simulink model "deteccao_2016_V7_somenteEHAs_comfiltro_"  (R2016a)
settings: Solver=FixedStepAuto  StartTime=72.65  StopTime=73.9  FixedStep=Ts  MaxStep=1e-7  RelTol=1e-4  AbsTol=1e-4
PreLoadFcn:
  | % -- Recommended Settings --
  | %
  | %  Simulink:
  | %      Solver: Ode23t
  | %      Relative tolerance = 1e-3
  | %       Max step size = 0.2
  | %
  | %  Powergui:
  |          Ts = 1e-07; % (discrete electrical model)
  | %
  | %  Control systems:
  |          Ts_control = 10*Ts; % (discrete control system)
  | %
  | % ----------------------------------
undefined symbols (not defined in the file or in its folder): C, L, R1, R2, sigbuilder_block
libraries: powerlib x92, dsparch4 x12, simulink x6, sps_avr x1, powerlib_meascontrol x1
(part 1 of 2)
settings Model: Creator=Joao  LastModifiedBy=Joao
settings DataIOCC: FinalStateName=xFinal_400_fixedstep  InitialState=xFinal_400_fixedstep  LimitDataPoints=on  SaveCompleteFinalSimState=on
settings DebuggingCC: UnconnectedInputMsg=none  UnconnectedOutputMsg=none  UnconnectedLineMsg=none  AllowSymbolicDim=off
settings ConfigComp: CovModelRefEnable=Off  CovSFcnEnable=off

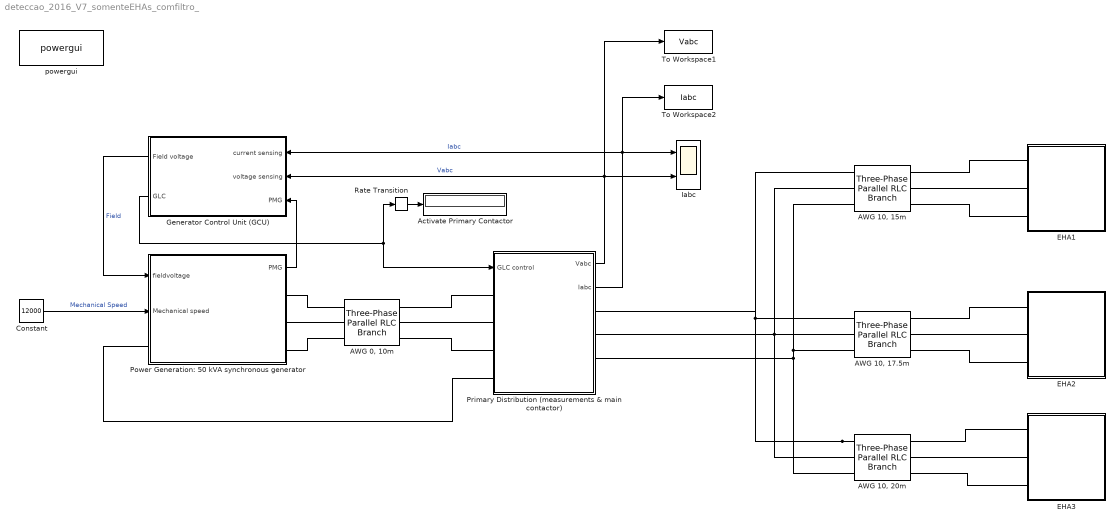
== system deteccao_2016_V7_somenteEHAs_comfiltro_ ==
  "AWG 0, 10m" : powerlib/Elements/Three-Phase Parallel RLC Branch  LConnTagsString=A|B|C  RConnTagsString=A|B|C  BranchType=RL  Resistance=0.00047*10  Inductance=0.2663e-06*10  Capacitance=0  Measurements=None
  "AWG 10, 15m" : powerlib/Elements/Three-Phase Parallel RLC Branch  LConnTagsString=A|B|C  RConnTagsString=A|B|C  BranchType=RL  Resistance=0.0036*15  Inductance=5.2869e-07*15  Capacitance=0  Measurements=None
  "AWG 10, 17.5m" : powerlib/Elements/Three-Phase Parallel RLC Branch  LConnTagsString=A|B|C  RConnTagsString=A|B|C  BranchType=RL  Resistance=0.0036*17.5  Inductance=5.2869e-07*17.5  Capacitance=0  Measurements=None
  "AWG 10, 20m" : powerlib/Elements/Three-Phase Parallel RLC Branch  LConnTagsString=A|B|C  RConnTagsString=A|B|C  BranchType=RL  Resistance=0.0036*20  Inductance=5.2869e-07*20  Capacitance=0  Measurements=None
  Activate Primary Contactor : Display
      settings: SampleTime=1e-2
  Constant : Constant  Value=12000
  EHA1 : Subsystem
  EHA2 : Subsystem
  EHA3 : Subsystem
  Generator Control Unit (GCU) : Subsystem
      mask Display: image(imread('power_aircraft_distribution_GCU.jpg','jpg'))
  Iabc : Scope  NumInputPorts=2
  Power Generation: 50 kVA synchronous generator : Subsystem
      mask Display: image(imread('power_aircraft_distribution_APU_Generator.jpg','jpg'))
  Primary Distribution (measurements & main contactor) : Subsystem
  Rate Transition : RateTransition  OutPortSampleTimeOpt=Inherit  OutPortSampleTime=Ts
  To Workspace1 : ToWorkspace  VariableName=Vabc  SaveFormat=Structure With Time  SampleTime=-1
  To Workspace2 : ToWorkspace  VariableName=Iabc  SaveFormat=Structure With Time  SampleTime=-1
  powergui : powerlib/powergui  Priority=1  SimulationMode=Continuous  SolverType=Tustin/Backward Euler (TBE)  SampleTime=Ts  frequency=60  SPID=on  DisableSnubberDevices=on  DisableRonSwitches=on  DisableVfSwitches=on  SwTol=0  DisplayEquations=off  Interpol=off  ExternalGateDelay=off  methode=off  Ts=100  FunctionMessages=on  echomessages=off  HookPort=off  EnableUseOfTLC=off  x0status=blocks  frequencyindice=0  Pbase=100e6  ErrMax=1e-4  Iterations=50  UnitsV=kV  UnitsW=MW  buscounter=0  RestoreLinks=warning  ResistiveCurrentMeasurement=off  Frange=[0:2:500]  Ylog=off  Xlog=on  ShowGrid=off  save=off  variable=ZData  structure=0  ZoomFFT=off  StartTime=0.0  cycles=1  DisplayStyle=1  fundamental=60  FreqAxis=off  MaxFrequency=1000  frequencyindicesteady=1  RmsSteady=1  display=off
  wires:
  Power Generation: 50 kVA synchronous generator/1(PMG) -> Generator Control Unit (GCU)/3(PMG)
  Generator Control Unit (GCU)/1(Field voltage) -> Power Generation: 50 kVA synchronous generator/1(fieldvoltage)  "Field"
  Primary Distribution (measurements & main contactor)/1(Vabc) -> Iabc/2, To Workspace1/1, Generator Control Unit (GCU)/2(voltage sensing)  "Vabc"
  Primary Distribution (measurements & main contactor)/2(Iabc) -> Generator Control Unit (GCU)/1(current sensing), To Workspace2/1, Iabc/1  "Iabc"
  Generator Control Unit (GCU)/2(GLC) -> Primary Distribution (measurements & main contactor)/1(GLC control), Rate Transition/1
  Constant/1 -> Power Generation: 50 kVA synchronous generator/2(Mechanical speed)  "Mechanical Speed"
  Rate Transition/1 -> Activate Primary Contactor/1
  connections:
  "AWG 10, 20m"/LConn1 -- "AWG 10, 15m"/LConn1 -- Primary Distribution (measurements & main contactor)/RConn1 -- "AWG 10, 17.5m"/LConn1
  "AWG 10, 17.5m"/LConn3 -- "AWG 10, 15m"/LConn3 -- "AWG 10, 20m"/LConn3 -- Primary Distribution (measurements & main contactor)/RConn3
  "AWG 10, 17.5m"/LConn2 -- "AWG 10, 15m"/LConn2 -- Primary Distribution (measurements & main contactor)/RConn2 -- "AWG 10, 20m"/LConn2
  "AWG 0, 10m"/RConn2 -- Primary Distribution (measurements & main contactor)/LConn2
  "AWG 0, 10m"/LConn2 -- Power Generation: 50 kVA synchronous generator/RConn2
  "AWG 0, 10m"/LConn1 -- Power Generation: 50 kVA synchronous generator/RConn1
  "AWG 0, 10m"/LConn3 -- Power Generation: 50 kVA synchronous generator/RConn3
  "AWG 0, 10m"/RConn1 -- Primary Distribution (measurements & main contactor)/LConn1
  "AWG 0, 10m"/RConn3 -- Primary Distribution (measurements & main contactor)/LConn3
  Power Generation: 50 kVA synchronous generator/LConn1 -- Primary Distribution (measurements & main contactor)/LConn4
  "AWG 10, 15m"/RConn1 -- EHA1/LConn1
  "AWG 10, 15m"/RConn2 -- EHA1/LConn2
  "AWG 10, 15m"/RConn3 -- EHA1/LConn3
  "AWG 10, 17.5m"/RConn1 -- EHA2/LConn1
  "AWG 10, 17.5m"/RConn2 -- EHA2/LConn2
  "AWG 10, 17.5m"/RConn3 -- EHA2/LConn3
  EHA3/LConn1 -- "AWG 10, 20m"/RConn1
  EHA3/LConn2 -- "AWG 10, 20m"/RConn2
  "AWG 10, 20m"/RConn3 -- EHA3/LConn3

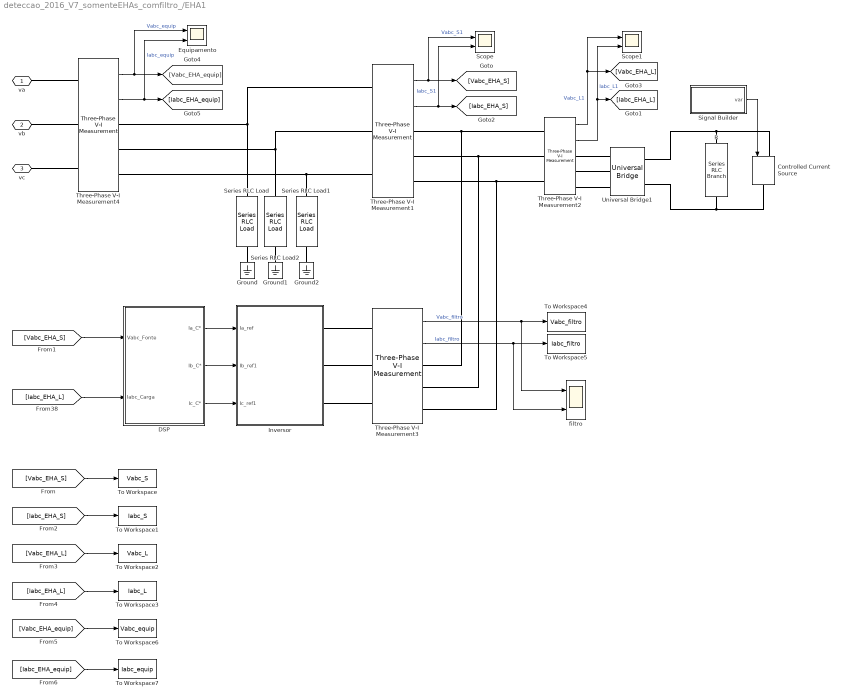
== system deteccao_2016_V7_somenteEHAs_comfiltro_/EHA1 ==
  Controlled Current Source : powerlib/Electrical Sources/Controlled Current Source  Initialize=on  Source_Type=AC  Amplitude=0  Phase=0  Frequency=0  Measurements=None
  DSP : Subsystem
  Equipamento : Scope  NumInputPorts=2
  Ground : powerlib/Elements/Ground  LConnTagsString=a
  Ground1 : powerlib/Elements/Ground  LConnTagsString=a
  Ground2 : powerlib/Elements/Ground  LConnTagsString=a
  Inversor : Subsystem
  R : powerlib/Elements/Series RLC Branch  LConnTagsString=__new0  RConnTagsString=__new0  BranchType=R  Resistance=10e3  Inductance=1e-3  SetiL0=off  InitialCurrent=0  Capacitance=1e-10  Setx0=off  InitialVoltage=0  Measurements=None
  Scope : Scope  NumInputPorts=2
  Scope1 : Scope  NumInputPorts=2
  Series RLC Load : powerlib/Elements/Series RLC Load  LConnTagsString=a  RConnTagsString=__new0  NominalVoltage=115  NominalFrequency=400  ActivePower=1  InductivePower=115^2*2*pi*400*C  CapacitivePower=0  Setx0=off  InitialVoltage=0  SetiL0=off  InitialCurrent=0  Measurements=None  LoadType=constant Z
  Series RLC Load1 : powerlib/Elements/Series RLC Load  LConnTagsString=a  RConnTagsString=__new0  NominalVoltage=115  NominalFrequency=400  ActivePower=1  InductivePower=115^2*2*pi*400*C  CapacitivePower=0  Setx0=off  InitialVoltage=0  SetiL0=off  InitialCurrent=0  Measurements=None  LoadType=constant Z
  Series RLC Load2 : powerlib/Elements/Series RLC Load  LConnTagsString=a  RConnTagsString=__new0  NominalVoltage=115  NominalFrequency=400  ActivePower=1  InductivePower=115^2*2*pi*400*C  CapacitivePower=0  Setx0=off  InitialVoltage=0  SetiL0=off  InitialCurrent=0  Measurements=None  LoadType=constant Z
  Signal Builder : Subsystem  Tag=STV Subsys  LoadFcn=sigbuilder_block('load');  StartFcn=sigbuilder_block('start');  StopFcn=sigbuilder_block('stop');  ClipboardFcn=sigbuilder_block('clipboard');  mask(Sigbuilder block){}
      mask help: Simulink:masks:SigbuilderBlock_MD
      mask init:
      | if ~strcmp(get_param(bdroot(gcbh),'SimulationStatus'),'stopped') tuvar = sigbuilder_block('maskInit'); end
      settings: CopyFcn=sigbuilder_block('copy');  DeleteFcn=sigbuilder_block('delete');  ModelCloseFcn=sigbuilder_block('modelClose');  PreSaveFcn=sigbuilder_block('preSave');  PauseFcn=sigbuilder_block('pause');  ContinueFcn=sigbuilder_block('continue');  NameChangeFcn=sigbuilder_block('namechange');  OpenFcn=sigbuilder_block('open',[437.6 199.2 550.4 400 ]);  CloseFcn=sigbuilder_block('close');
      mask Display: plot(0, 0, 100, 100,[2, 2, 32, 32, 2], [68, 8, 8, 68, 68],[32, 2], [38, 38], [32, 19, 2],[53, 60, 44], [32, 17, 17, 2],[16, 16, 31, 31]);txt = getActiveGroup(gcbh);text(2, 100, txt,'verticalAlignment', 'top');
  Three-Phase V-I Measurement{1..4} (4 alike) : powerlib/Measurements/Three-Phase V-I Measurement  VoltageMeasurement=phase-to-ground  SetLabelV=off  LabelV=Vabc_EHA1_S  Vpu=off  VpuLL=off  CurrentMeasurement=yes  SetLabelI=off  LabelI=Iabc_EHA1_S  Ipu=off  Pbase=100e6  Vbase=500e3  OutputType=Complex  PhasorSimulation=off  PSBequivalent=0
  To Workspace : ToWorkspace  VariableName=Vabc_S  SaveFormat=Structure With Time  SampleTime=-1
  To Workspace1 : ToWorkspace  VariableName=Iabc_S  SaveFormat=Structure With Time  SampleTime=-1
  To Workspace2 : ToWorkspace  VariableName=Vabc_L  SaveFormat=Structure With Time  SampleTime=-1
  To Workspace3 : ToWorkspace  VariableName=Iabc_L  SaveFormat=Structure With Time  SampleTime=-1
  To Workspace4 : ToWorkspace  VariableName=Vabc_filtro  SaveFormat=Structure With Time  SampleTime=-1
  To Workspace5 : ToWorkspace  VariableName=Iabc_filtro  SaveFormat=Structure With Time  SampleTime=-1
  To Workspace6 : ToWorkspace  VariableName=Vabc_equip  SaveFormat=Structure With Time  SampleTime=-1
  To Workspace7 : ToWorkspace  VariableName=Iabc_equip  SaveFormat=Structure With Time  SampleTime=-1
  Universal Bridge1 : powerlib/Power Electronics/Universal Bridge  Arms=3  SnubberResistance=1e5  SnubberCapacitance=inf  Device=Diodes  Ron=1e-9  Lon=0  ForwardVoltages="[  0  0  ]"  ForwardVoltage=0  GTOparameters=[ 10e-6 , 20e-6 ]  IGBTparameters=[ 1e-6 , 2e-6 ]  Measurements=None  Measurements_2=None  converterType=Rectifier
  filtro : Scope  NumInputPorts=2
  va : PMIOPort  Port=1  Side=Left
  vb : PMIOPort  Port=2  Side=Left
  vc : PMIOPort  Port=3  Side=Left
  wires:
  Three-Phase V-I Measurement1/1 -> [Vabc_EHA_S], Scope/1  "Vabc_S1"
  Three-Phase V-I Measurement1/2 -> [Iabc_EHA_S], Scope/2  "Iabc_S1"
  Three-Phase V-I Measurement2/1 -> [Vabc_EHA_L], Scope1/1  "Vabc_L1"
  Three-Phase V-I Measurement2/2 -> [Iabc_EHA_L], Scope1/2  "Iabc_L1"
  [Vabc_EHA_S] -> DSP/1(Vabc_Fonte)
  [Iabc_EHA_L] -> DSP/2(Iabc_Carga)
  DSP/1(Ia_C*) -> Inversor/1(Ia_ref)
  DSP/2(Ib_C*) -> Inversor/2(Ib_ref1)
  DSP/3(Ic_C*) -> Inversor/3(Ic_ref1)
  [Vabc_EHA_S] -> To Workspace/1
  [Iabc_EHA_S] -> To Workspace1/1
  [Vabc_EHA_L] -> To Workspace2/1
  [Iabc_EHA_L] -> To Workspace3/1
  Signal Builder/1(var) -> Controlled Current Source/1
  Three-Phase V-I Measurement3/1 -> filtro/1, To Workspace4/1  "Vabc_filtro"
  Three-Phase V-I Measurement3/2 -> filtro/2, To Workspace5/1  "Iabc_filtro"
  Three-Phase V-I Measurement4/1 -> [Vabc_EHA_equip], Equipamento/1  "Vabc_equip"
  Three-Phase V-I Measurement4/2 -> [Iabc_EHA_equip], Equipamento/2  "Iabc_equip"
  [Vabc_EHA_equip] -> To Workspace6/1
  [Iabc_EHA_equip] -> To Workspace7/1
  connections:
  Controlled Current Source/LConn1 -- R/LConn1 -- Universal Bridge1/RConn1
  Controlled Current Source/RConn1 -- R/RConn1 -- Universal Bridge1/RConn2
  Three-Phase V-I Measurement2/RConn2 -- Universal Bridge1/LConn2
  Three-Phase V-I Measurement2/RConn1 -- Universal Bridge1/LConn1
  Three-Phase V-I Measurement2/RConn3 -- Universal Bridge1/LConn3
  Three-Phase V-I Measurement2/LConn3 -- Three-Phase V-I Measurement3/RConn3 -- Three-Phase V-I Measurement1/RConn3
  Three-Phase V-I Measurement1/RConn1 -- Three-Phase V-I Measurement3/RConn1 -- Three-Phase V-I Measurement2/LConn1
  Three-Phase V-I Measurement1/RConn2 -- Three-Phase V-I Measurement3/RConn2 -- Three-Phase V-I Measurement2/LConn2
  Series RLC Load2/LConn1 -- Three-Phase V-I Measurement4/RConn2 -- Three-Phase V-I Measurement1/LConn2
  Series RLC Load1/LConn1 -- Three-Phase V-I Measurement4/RConn3 -- Three-Phase V-I Measurement1/LConn3
  Series RLC Load/LConn1 -- Three-Phase V-I Measurement4/RConn1 -- Three-Phase V-I Measurement1/LConn1
  Three-Phase V-I Measurement3/LConn2 -- Inversor/RConn2
  Three-Phase V-I Measurement3/LConn1 -- Inversor/RConn1
  Three-Phase V-I Measurement3/LConn3 -- Inversor/RConn3
  Ground/LConn1 -- Series RLC Load/RConn1
  Ground2/LConn1 -- Series RLC Load1/RConn1
  Ground1/LConn1 -- Series RLC Load2/RConn1
  vc/RConn1 -- Three-Phase V-I Measurement4/LConn3
  vb/RConn1 -- Three-Phase V-I Measurement4/LConn2
  va/RConn1 -- Three-Phase V-I Measurement4/LConn1

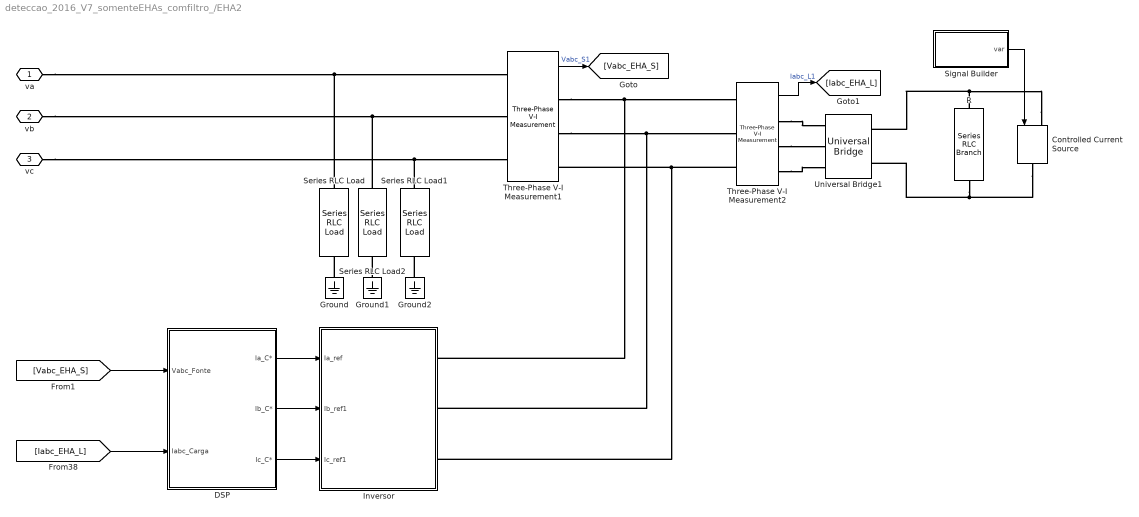
== system deteccao_2016_V7_somenteEHAs_comfiltro_/EHA2 ==
  Controlled Current Source : powerlib/Electrical Sources/Controlled Current Source  Initialize=on  Source_Type=AC  Amplitude=0  Phase=0  Frequency=0  Measurements=None
  DSP : Subsystem
  Ground : powerlib/Elements/Ground  LConnTagsString=a
  Ground1 : powerlib/Elements/Ground  LConnTagsString=a
  Ground2 : powerlib/Elements/Ground  LConnTagsString=a
  Inversor : Subsystem
  R : powerlib/Elements/Series RLC Branch  LConnTagsString=__new0  RConnTagsString=__new0  BranchType=R  Resistance=2e3  Inductance=1e-3  SetiL0=off  InitialCurrent=0  Capacitance=1e-10  Setx0=off  InitialVoltage=0  Measurements=None
  Series RLC Load : powerlib/Elements/Series RLC Load  LConnTagsString=a  RConnTagsString=__new0  NominalVoltage=115  NominalFrequency=400  ActivePower=1  InductivePower=115^2*2*pi*400*C  CapacitivePower=0  Setx0=off  InitialVoltage=0  SetiL0=off  InitialCurrent=0  Measurements=None  LoadType=constant Z
  Series RLC Load1 : powerlib/Elements/Series RLC Load  LConnTagsString=a  RConnTagsString=__new0  NominalVoltage=115  NominalFrequency=400  ActivePower=1  InductivePower=115^2*2*pi*400*C  CapacitivePower=0  Setx0=off  InitialVoltage=0  SetiL0=off  InitialCurrent=0  Measurements=None  LoadType=constant Z
  Series RLC Load2 : powerlib/Elements/Series RLC Load  LConnTagsString=a  RConnTagsString=__new0  NominalVoltage=115  NominalFrequency=400  ActivePower=1  InductivePower=115^2*2*pi*400*C  CapacitivePower=0  Setx0=off  InitialVoltage=0  SetiL0=off  InitialCurrent=0  Measurements=None  LoadType=constant Z
  Signal Builder : Subsystem  Tag=STV Subsys  LoadFcn=sigbuilder_block('load');  StartFcn=sigbuilder_block('start');  StopFcn=sigbuilder_block('stop');  ClipboardFcn=sigbuilder_block('clipboard');  mask(Sigbuilder block){}
      mask help: Simulink:masks:SigbuilderBlock_MD
      mask init:
      | if ~strcmp(get_param(bdroot(gcbh),'SimulationStatus'),'stopped') tuvar = sigbuilder_block('maskInit'); end
      settings: CopyFcn=sigbuilder_block('copy');  DeleteFcn=sigbuilder_block('delete');  ModelCloseFcn=sigbuilder_block('modelClose');  PreSaveFcn=sigbuilder_block('preSave');  PauseFcn=sigbuilder_block('pause');  ContinueFcn=sigbuilder_block('continue');  NameChangeFcn=sigbuilder_block('namechange');  OpenFcn=sigbuilder_block('open',[437.6 199.2 550.4 400 ]);  CloseFcn=sigbuilder_block('close');
      mask Display: plot(0, 0, 100, 100,[2, 2, 32, 32, 2], [68, 8, 8, 68, 68],[32, 2], [38, 38], [32, 19, 2],[53, 60, 44], [32, 17, 17, 2],[16, 16, 31, 31]);txt = getActiveGroup(gcbh);text(2, 100, txt,'verticalAlignment', 'top');
  Three-Phase V-I Measurement1 : powerlib/Measurements/Three-Phase V-I Measurement  VoltageMeasurement=phase-to-ground  SetLabelV=off  LabelV=Vabc_EHA1_S  Vpu=off  VpuLL=off  CurrentMeasurement=no  SetLabelI=off  LabelI=Iabc_EHA1_S  Ipu=off  Pbase=100e6  Vbase=500e3  OutputType=Complex  PhasorSimulation=off  PSBequivalent=0
  Three-Phase V-I Measurement2 : powerlib/Measurements/Three-Phase V-I Measurement  VoltageMeasurement=no  SetLabelV=off  LabelV=Vabc_EHA1_S  Vpu=off  VpuLL=off  CurrentMeasurement=yes  SetLabelI=off  LabelI=Iabc_EHA1_S  Ipu=off  Pbase=100e6  Vbase=500e3  OutputType=Complex  PhasorSimulation=off  PSBequivalent=0
  Universal Bridge1 : powerlib/Power Electronics/Universal Bridge  Arms=3  SnubberResistance=1e5  SnubberCapacitance=inf  Device=Diodes  Ron=1e-9  Lon=0  ForwardVoltages="[  0  0  ]"  ForwardVoltage=0  GTOparameters=[ 10e-6 , 20e-6 ]  IGBTparameters=[ 1e-6 , 2e-6 ]  Measurements=None  Measurements_2=None  converterType=Rectifier
  va : PMIOPort  Port=1  Side=Left
  vb : PMIOPort  Port=2  Side=Left
  vc : PMIOPort  Port=3  Side=Left
  wires:
  Three-Phase V-I Measurement1/1 -> [Vabc_EHA_S]  "Vabc_S1"
  Three-Phase V-I Measurement2/1 -> [Iabc_EHA_L]  "Iabc_L1"
  [Vabc_EHA_S] -> DSP/1(Vabc_Fonte)
  [Iabc_EHA_L] -> DSP/2(Iabc_Carga)
  DSP/1(Ia_C*) -> Inversor/1(Ia_ref)
  DSP/2(Ib_C*) -> Inversor/2(Ib_ref1)
  DSP/3(Ic_C*) -> Inversor/3(Ic_ref1)
  Signal Builder/1(var) -> Controlled Current Source/1
  connections:
  Controlled Current Source/LConn1 -- R/LConn1 -- Universal Bridge1/RConn1
  Controlled Current Source/RConn1 -- R/RConn1 -- Universal Bridge1/RConn2
  Three-Phase V-I Measurement2/RConn2 -- Universal Bridge1/LConn2
  Three-Phase V-I Measurement2/RConn1 -- Universal Bridge1/LConn1
  Three-Phase V-I Measurement2/RConn3 -- Universal Bridge1/LConn3
  vb/RConn1 -- Series RLC Load2/LConn1 -- Three-Phase V-I Measurement1/LConn2
  vc/RConn1 -- Series RLC Load1/LConn1 -- Three-Phase V-I Measurement1/LConn3
  va/RConn1 -- Series RLC Load/LConn1 -- Three-Phase V-I Measurement1/LConn1
  Three-Phase V-I Measurement1/RConn2 -- Inversor/RConn2 -- Three-Phase V-I Measurement2/LConn2
  Three-Phase V-I Measurement1/RConn1 -- Inversor/RConn1 -- Three-Phase V-I Measurement2/LConn1
  Three-Phase V-I Measurement2/LConn3 -- Three-Phase V-I Measurement1/RConn3 -- Inversor/RConn3
  Ground1/LConn1 -- Series RLC Load2/RConn1
  Ground/LConn1 -- Series RLC Load/RConn1
  Ground2/LConn1 -- Series RLC Load1/RConn1

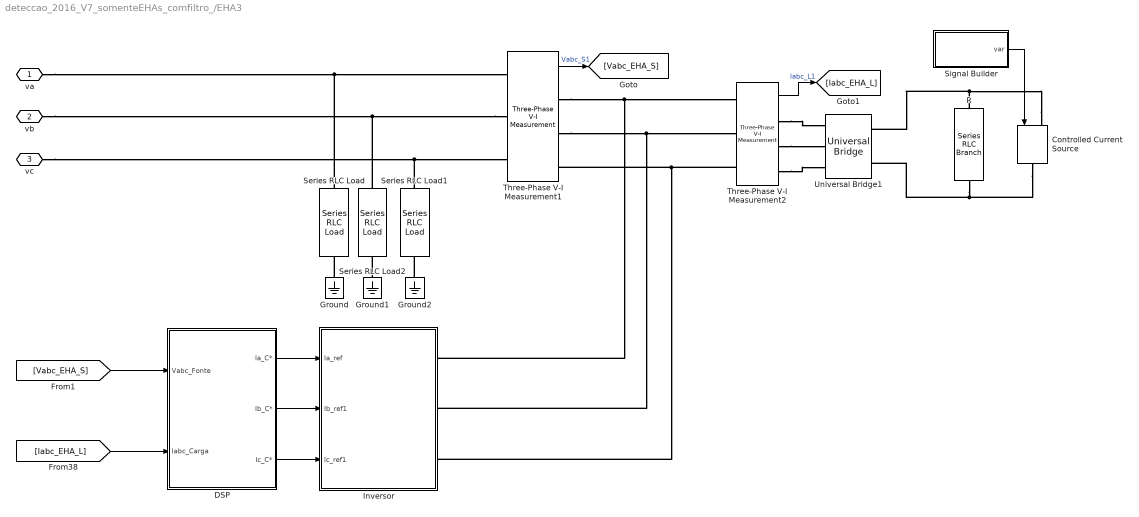
== system deteccao_2016_V7_somenteEHAs_comfiltro_/EHA3 ==
  Controlled Current Source : powerlib/Electrical Sources/Controlled Current Source  Initialize=on  Source_Type=AC  Amplitude=0  Phase=0  Frequency=0  Measurements=None
  DSP : Subsystem
  Ground : powerlib/Elements/Ground  LConnTagsString=a
  Ground1 : powerlib/Elements/Ground  LConnTagsString=a
  Ground2 : powerlib/Elements/Ground  LConnTagsString=a
  Inversor : Subsystem
  R : powerlib/Elements/Series RLC Branch  LConnTagsString=__new0  RConnTagsString=__new0  BranchType=R  Resistance=2e3  Inductance=1e-3  SetiL0=off  InitialCurrent=0  Capacitance=1e-10  Setx0=off  InitialVoltage=0  Measurements=None
  Series RLC Load : powerlib/Elements/Series RLC Load  LConnTagsString=a  RConnTagsString=__new0  NominalVoltage=115  NominalFrequency=400  ActivePower=1  InductivePower=115^2*2*pi*400*C  CapacitivePower=0  Setx0=off  InitialVoltage=0  SetiL0=off  InitialCurrent=0  Measurements=None  LoadType=constant Z
  Series RLC Load1 : powerlib/Elements/Series RLC Load  LConnTagsString=a  RConnTagsString=__new0  NominalVoltage=115  NominalFrequency=400  ActivePower=1  InductivePower=115^2*2*pi*400*C  CapacitivePower=0  Setx0=off  InitialVoltage=0  SetiL0=off  InitialCurrent=0  Measurements=None  LoadType=constant Z
  Series RLC Load2 : powerlib/Elements/Series RLC Load  LConnTagsString=a  RConnTagsString=__new0  NominalVoltage=115  NominalFrequency=400  ActivePower=1  InductivePower=115^2*2*pi*400*C  CapacitivePower=0  Setx0=off  InitialVoltage=0  SetiL0=off  InitialCurrent=0  Measurements=None  LoadType=constant Z
  Signal Builder : Subsystem  Tag=STV Subsys  LoadFcn=sigbuilder_block('load');  StartFcn=sigbuilder_block('start');  StopFcn=sigbuilder_block('stop');  ClipboardFcn=sigbuilder_block('clipboard');  mask(Sigbuilder block){}
      mask help: Simulink:masks:SigbuilderBlock_MD
      mask init:
      | if ~strcmp(get_param(bdroot(gcbh),'SimulationStatus'),'stopped') tuvar = sigbuilder_block('maskInit'); end
      settings: CopyFcn=sigbuilder_block('copy');  DeleteFcn=sigbuilder_block('delete');  ModelCloseFcn=sigbuilder_block('modelClose');  PreSaveFcn=sigbuilder_block('preSave');  PauseFcn=sigbuilder_block('pause');  ContinueFcn=sigbuilder_block('continue');  NameChangeFcn=sigbuilder_block('namechange');  OpenFcn=sigbuilder_block('open',[437.6 199.2 550.4 400 ]);  CloseFcn=sigbuilder_block('close');
      mask Display: plot(0, 0, 100, 100,[2, 2, 32, 32, 2], [68, 8, 8, 68, 68],[32, 2], [38, 38], [32, 19, 2],[53, 60, 44], [32, 17, 17, 2],[16, 16, 31, 31]);txt = getActiveGroup(gcbh);text(2, 100, txt,'verticalAlignment', 'top');
  Three-Phase V-I Measurement1 : powerlib/Measurements/Three-Phase V-I Measurement  VoltageMeasurement=phase-to-ground  SetLabelV=off  LabelV=Vabc_EHA1_S  Vpu=off  VpuLL=off  CurrentMeasurement=no  SetLabelI=off  LabelI=Iabc_EHA1_S  Ipu=off  Pbase=100e6  Vbase=500e3  OutputType=Complex  PhasorSimulation=off  PSBequivalent=0
  Three-Phase V-I Measurement2 : powerlib/Measurements/Three-Phase V-I Measurement  VoltageMeasurement=no  SetLabelV=off  LabelV=Vabc_EHA1_S  Vpu=off  VpuLL=off  CurrentMeasurement=yes  SetLabelI=off  LabelI=Iabc_EHA1_S  Ipu=off  Pbase=100e6  Vbase=500e3  OutputType=Complex  PhasorSimulation=off  PSBequivalent=0
  Universal Bridge1 : powerlib/Power Electronics/Universal Bridge  Arms=3  SnubberResistance=1e5  SnubberCapacitance=inf  Device=Diodes  Ron=1e-9  Lon=0  ForwardVoltages="[  0  0  ]"  ForwardVoltage=0  GTOparameters=[ 10e-6 , 20e-6 ]  IGBTparameters=[ 1e-6 , 2e-6 ]  Measurements=None  Measurements_2=None  converterType=Rectifier
  va : PMIOPort  Port=1  Side=Left
  vb : PMIOPort  Port=2  Side=Left
  vc : PMIOPort  Port=3  Side=Left
  wires:
  Three-Phase V-I Measurement1/1 -> [Vabc_EHA_S]  "Vabc_S1"
  Three-Phase V-I Measurement2/1 -> [Iabc_EHA_L]  "Iabc_L1"
  [Vabc_EHA_S] -> DSP/1(Vabc_Fonte)
  [Iabc_EHA_L] -> DSP/2(Iabc_Carga)
  DSP/1(Ia_C*) -> Inversor/1(Ia_ref)
  DSP/2(Ib_C*) -> Inversor/2(Ib_ref1)
  DSP/3(Ic_C*) -> Inversor/3(Ic_ref1)
  Signal Builder/1(var) -> Controlled Current Source/1
  connections:
  Controlled Current Source/LConn1 -- R/LConn1 -- Universal Bridge1/RConn1
  Controlled Current Source/RConn1 -- R/RConn1 -- Universal Bridge1/RConn2
  Three-Phase V-I Measurement2/RConn2 -- Universal Bridge1/LConn2
  Three-Phase V-I Measurement2/RConn1 -- Universal Bridge1/LConn1
  Three-Phase V-I Measurement2/RConn3 -- Universal Bridge1/LConn3
  Three-Phase V-I Measurement1/LConn2 -- Series RLC Load2/LConn1 -- vb/RConn1
  vc/RConn1 -- Series RLC Load1/LConn1 -- Three-Phase V-I Measurement1/LConn3
  va/RConn1 -- Series RLC Load/LConn1 -- Three-Phase V-I Measurement1/LConn1
  Three-Phase V-I Measurement1/RConn2 -- Three-Phase V-I Measurement2/LConn2 -- Inversor/RConn2
  Three-Phase V-I Measurement1/RConn1 -- Three-Phase V-I Measurement2/LConn1 -- Inversor/RConn1
  Three-Phase V-I Measurement2/LConn3 -- Inversor/RConn3 -- Three-Phase V-I Measurement1/RConn3
  Ground1/LConn1 -- Series RLC Load2/RConn1
  Ground/LConn1 -- Series RLC Load/RConn1
  Ground2/LConn1 -- Series RLC Load1/RConn1

== system deteccao_2016_V7_somenteEHAs_comfiltro_/Generator Control Unit (GCU) ==
  current sensing : Inport
  voltage sensing : Inport  Port=2
  PMG : Inport  Port=3
  Demux : Demux  Outputs=3
  Excitation System : sps_avr/Excitation System  tr=20e-3  reg=[ 300, 0.001 ]  exc=[ 1, 0 ]  tgr=[ 0, 0 ]  damp=[ 0.001, 0.1 ]  sat=[ 0, 0 ]  lim=[ -2, 2, 0 ]  v0=[1 0]
  Gain : Gain  Gain=2
  Integrator : Integrator
  PU_SI : Gain  Gain=200
  Rad_Rpm : Gain  Gain=30/pi
  Relay : Relay  OnSwitchValue=9000  OffSwitchValue=8900
  SI_PU : Gain  Gain=1/(115*sqrt(2))
  Terminator1 : Terminator
  Terminator2 : Terminator
  Vref : Constant
  abc to dq0 : powerlib_meascontrol/Transformations/abc to dq0  Alignment=90 degrees behind phase A axis
  threshold3 : Constant  Value=0
  Field voltage : Outport
  GLC : Outport  Port=2
  wires:
  Relay/1 -> GLC/1
  Demux/3 -> Terminator2/1
  current sensing/1 -> Terminator1/1
  threshold3/1 -> Excitation System/4
  Vref/1 -> Excitation System/1
  Rad_Rpm/1 -> Relay/1
  PU_SI/1 -> Field voltage/1
  Excitation System/1 -> PU_SI/1
  SI_PU/1 -> abc to dq0/1
  Demux/2 -> Excitation System/3
  Demux/1 -> Excitation System/2
  abc to dq0/1 -> Demux/1
  Integrator/1 -> Gain/1
  voltage sensing/1 -> SI_PU/1
  PMG/1 -> Rad_Rpm/1, Integrator/1
  Gain/1 -> abc to dq0/2

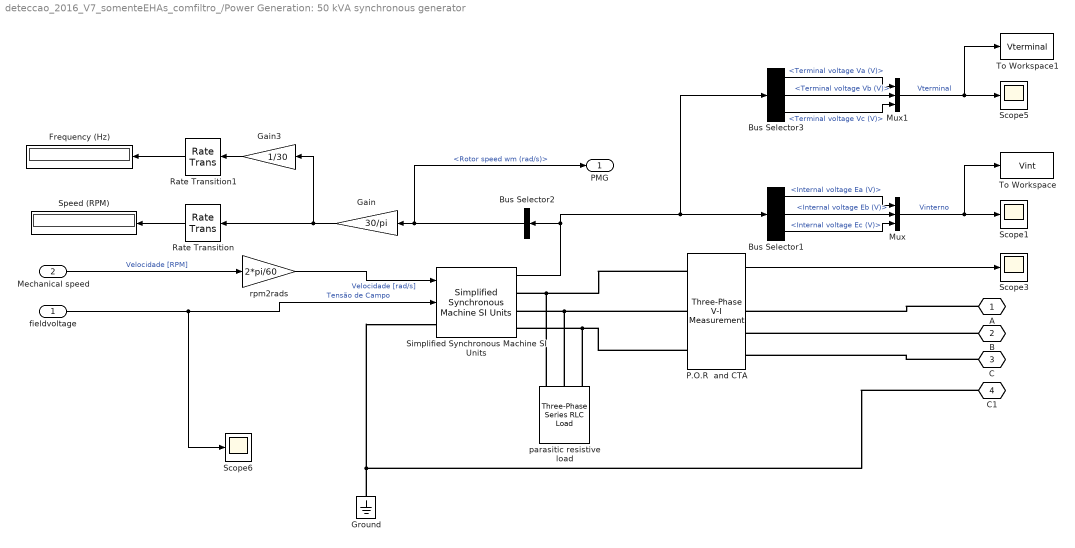
== system deteccao_2016_V7_somenteEHAs_comfiltro_/Power Generation: 50 kVA synchronous generator ==
  fieldvoltage : Inport
  Mechanical speed : Inport  Port=2
  Bus Selector1 : BusSelector  OutputSignals=Internal voltage Ea (V),Internal voltage Eb (V),Internal voltage Ec (V)
  Bus Selector2 : BusSelector  OutputSignals=Rotor speed wm (rad/s)
  Bus Selector3 : BusSelector  OutputSignals=Terminal voltage Va (V),Terminal voltage Vb (V),Terminal voltage Vc (V)
  Frequency (Hz) : Display
      settings: SampleTime=1e-2
  Gain : Gain  Gain=30/pi
  Gain3 : Gain  Gain=1/30
  Ground : powerlib/Elements/Ground  LConnTagsString=a
  Mux : Mux  Inputs=3
  Mux1 : Mux  Inputs=3
  P.O.R  and CTA : powerlib/Measurements/Three-Phase V-I Measurement  VoltageMeasurement=phase-to-ground  SetLabelV=off  LabelV=Vabc  Vpu=off  VpuLL=off  CurrentMeasurement=yes  SetLabelI=off  LabelI=Iabc  Ipu=off  Pbase=100e6  Vbase=500e3  OutputType=Complex  PhasorSimulation=off  PSBequivalent=0
  Rate Transition : RateTransition  OutPortSampleTimeOpt=Inherit  OutPortSampleTime=Ts
  Rate Transition1 : RateTransition  OutPortSampleTimeOpt=Inherit  OutPortSampleTime=Ts
  Scope{1,3,5..6} (4 alike) : Scope
  Simplified Synchronous Machine SI Units : powerlib/Machines/Simplified Synchronous Machine SI Units  ConnectionType=4-wire Y  MechanicalLoad=Speed w  MeasurementBus=off  NominalParameters=[50e3 200 400]  Mechanical=[0.02 0 2]  InternalRL="[0.0404  0.09204e-3]"  InitialConditions=[-99,0 0,0,0 0,0,0]  Units=1  LoadFlowParameters=[1,0,0,0,0]  TsPowergui=0  TsBlock=Ts  BusType=PV  Pref=0  Qref=0  Qmin=-inf  Qmax=+inf  PLF=0  QLF=0
  Speed (RPM) : Display
      settings: SampleTime=1e-2
  To Workspace : ToWorkspace  VariableName=Vint  SaveFormat=Structure With Time  SampleTime=-1
  To Workspace1 : ToWorkspace  VariableName=Vterminal  SaveFormat=Structure With Time  SampleTime=-1
  parasitic resistive load : powerlib/Elements/Three-Phase Series RLC Load  LConnTagsString=A|B|C  Configuration=Y (grounded)  NominalVoltage=200  Vabc=[1e3 1e3 1e3]  Vabcp=[1e3 1e3 1e3]  NominalFrequency=400  UnbalancedPower=off  ActivePower=5000  InductivePower=0  CapacitivePower=0  Pabc=[10e3 9e3 11e3]  QLabc=[100 90 110]  QCabc=[100 90 110]  Pabcp=[10e3 9e3 11e3]  QLabcp=[100 90 110]  QCabcp=[100 90 110]  Measurements=None  LoadType=constant Z
  rpm2rads : Gain  Gain=2*pi/60
  A : PMIOPort  Tag=PMCPort  Port=1  Side=Right
  B : PMIOPort  Tag=PMCPort  Port=2  Side=Right
  C : PMIOPort  Tag=PMCPort  Port=3  Side=Right
  C1 : PMIOPort  Tag=PMCPort  Port=4  Side=Left
  PMG : Outport
  wires:
  Simplified Synchronous Machine SI Units/1 -> Bus Selector3/1, Bus Selector1/1, Bus Selector2/1
  fieldvoltage/1 -> Scope6/1, Simplified Synchronous Machine SI Units/2  "Tensão de Campo"
  Bus Selector2/1 -> PMG/1, Gain/1  "<Rotor speed wm (rad/s)>"
  Gain/1 -> Gain3/1, Rate Transition/1
  Gain3/1 -> Rate Transition1/1
  Mechanical speed/1 -> rpm2rads/1  "Velocidade [RPM]"
  rpm2rads/1 -> Simplified Synchronous Machine SI Units/1  "Velocidade [rad/s]"
  Rate Transition/1 -> Speed (RPM)/1
  Rate Transition1/1 -> Frequency (Hz)/1
  Bus Selector1/2 -> Mux/2  "<Internal voltage Eb (V)>"
  Bus Selector1/3 -> Mux/3  "<Internal voltage Ec (V)>"
  Bus Selector1/1 -> Mux/1  "<Internal voltage Ea (V)>"
  Mux/1 -> Scope1/1, To Workspace/1  "Vinterno"
  P.O.R  and CTA/1 -> Scope3/1
  Bus Selector3/2 -> Mux1/2  "<Terminal voltage Vb (V)>"
  Bus Selector3/3 -> Mux1/3  "<Terminal voltage Vc (V)>"
  Bus Selector3/1 -> Mux1/1  "<Terminal voltage Va (V)>"
  Mux1/1 -> To Workspace1/1, Scope5/1  "Vterminal"
  connections:
  Ground/LConn1 -- C1/RConn1 -- Simplified Synchronous Machine SI Units/LConn1
  P.O.R  and CTA/LConn1 -- parasitic resistive load/LConn1 -- Simplified Synchronous Machine SI Units/RConn1
  P.O.R  and CTA/LConn2 -- parasitic resistive load/LConn2 -- Simplified Synchronous Machine SI Units/RConn2
  P.O.R  and CTA/LConn3 -- parasitic resistive load/LConn3 -- Simplified Synchronous Machine SI Units/RConn3
  A/RConn1 -- P.O.R  and CTA/RConn1
  B/RConn1 -- P.O.R  and CTA/RConn2
  C/RConn1 -- P.O.R  and CTA/RConn3

== system deteccao_2016_V7_somenteEHAs_comfiltro_/Primary Distribution (measurements & main contactor) ==
  note: Primary Distribution
  GLC control : Inport
  Contactor : Subsystem
  Current Measurement : powerlib/Measurements/Current Measurement  PhasorSimulation=off  OutputType=Complex  PSBequivalent=0
  Data Type Conversion : DataTypeConversion
  P.O.R  and CTA : powerlib/Measurements/Three-Phase V-I Measurement  VoltageMeasurement=phase-to-ground  SetLabelV=off  LabelV=Vabc  Vpu=off  VpuLL=off  CurrentMeasurement=yes  SetLabelI=off  LabelI=Iabc  Ipu=off  Pbase=100e6  Vbase=500e3  OutputType=Complex  PhasorSimulation=off  PSBequivalent=0
  Scope : Scope
  in_a : PMIOPort  Port=1  Side=Left
  in_b : PMIOPort  Port=2  Side=Left
  in_c : PMIOPort  Port=3  Side=Left
  out_a : PMIOPort  Port=4  Side=Right
  out_b : PMIOPort  Port=5  Side=Right
  out_c : PMIOPort  Port=6  Side=Right
  in_c1 : PMIOPort  Port=7  Side=Left
  out_c1 : PMIOPort  Port=8  Side=Right
  Vabc : Outport
  Iabc : Outport  Port=2
  wires:
  GLC control/1 -> Data Type Conversion/1
  P.O.R  and CTA/1 -> Vabc/1
  P.O.R  and CTA/2 -> Iabc/1
  Data Type Conversion/1 -> Contactor/1(com)
  Current Measurement/1 -> Scope/1
  connections:
  in_a/RConn1 -- P.O.R  and CTA/LConn1
  in_b/RConn1 -- P.O.R  and CTA/LConn2
  in_c/RConn1 -- P.O.R  and CTA/LConn3
  P.O.R  and CTA/RConn1 -- Contactor/LConn1
  P.O.R  and CTA/RConn2 -- Contactor/LConn2
  P.O.R  and CTA/RConn3 -- Contactor/LConn3
  Contactor/RConn1 -- out_a/RConn1
  out_b/RConn1 -- Contactor/RConn2
  Contactor/RConn3 -- out_c/RConn1
  Current Measurement/LConn1 -- in_c1/RConn1
  Current Measurement/RConn1 -- out_c1/RConn1

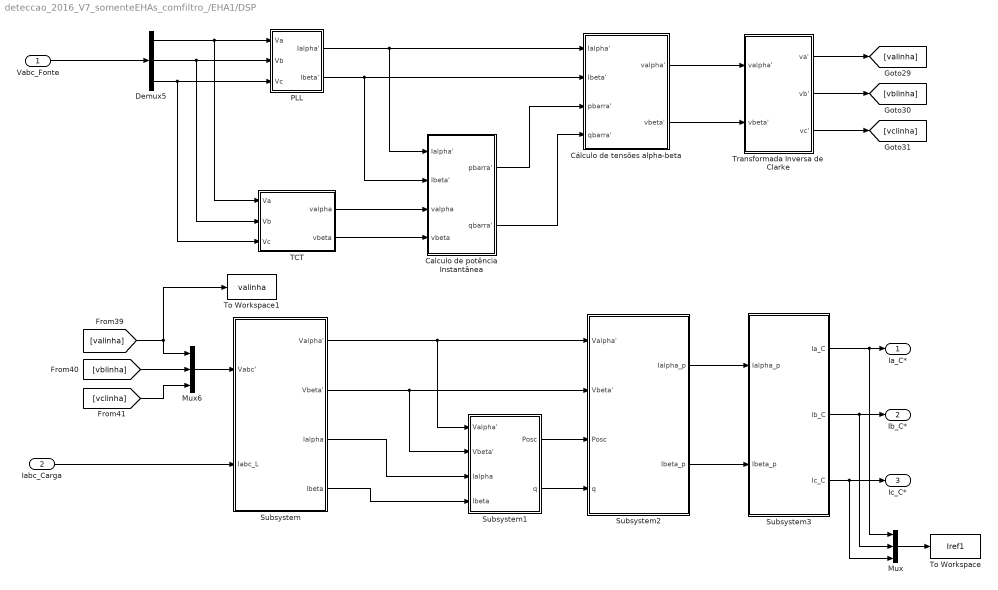
== system deteccao_2016_V7_somenteEHAs_comfiltro_/EHA1/DSP ==
  Vabc_Fonte : Inport
  Iabc_Carga : Inport  Port=2
  Calculo de potência Instantânea : Subsystem
  Cálculo de tensões alpha-beta : Subsystem
  Demux5 : Demux  Outputs=3
  Mux : Mux  Inputs=3
  Mux6 : Mux  Inputs=3
  PLL : Subsystem
  Subsystem : Subsystem
  Subsystem1 : Subsystem
  Subsystem2 : Subsystem
  Subsystem3 : Subsystem
  TCT : Subsystem
  To Workspace : ToWorkspace  VariableName=Iref1  SaveFormat=Structure With Time  SampleTime=-1
  To Workspace1 : ToWorkspace  VariableName=valinha  SaveFormat=Structure With Time  SampleTime=-1
  Transformada Inversa de Clarke : Subsystem
  Ia_C* : Outport
  Ib_C* : Outport  Port=2
  Ic_C* : Outport  Port=3
  wires:
  Vabc_Fonte/1 -> Demux5/1
  Demux5/1 -> PLL/1(Va), TCT/1(Va)
  Demux5/2 -> PLL/2(Vb), TCT/2(Vb)
  Demux5/3 -> PLL/3(Vc), TCT/3(Vc)
  TCT/1(valpha) -> Calculo de potência Instantânea/3(valpha)
  TCT/2(vbeta) -> Calculo de potência Instantânea/4(vbeta)
  Calculo de potência Instantânea/2(qbarra') -> Cálculo de tensões alpha-beta/4(qbarra')
  PLL/1(Ialpha') -> Calculo de potência Instantânea/1(Ialpha'), Cálculo de tensões alpha-beta/1(Ialpha')
  PLL/2(Ibeta') -> Calculo de potência Instantânea/2(Ibeta'), Cálculo de tensões alpha-beta/2(Ibeta')
  Calculo de potência Instantânea/1(pbarra') -> Cálculo de tensões alpha-beta/3(pbarra')
  Cálculo de tensões alpha-beta/1(valpha') -> Transformada Inversa de Clarke/1(valpha')
  Cálculo de tensões alpha-beta/2(vbeta') -> Transformada Inversa de Clarke/2(vbeta')
  Transformada Inversa de Clarke/1(va') -> [valinha]
  Transformada Inversa de Clarke/2(vb') -> [vblinha]
  Transformada Inversa de Clarke/3(vc') -> [vclinha]
  [valinha] -> Mux6/1, To Workspace1/1
  [vblinha] -> Mux6/2
  [vclinha] -> Mux6/3
  Mux6/1 -> Subsystem/1(Vabc')
  Iabc_Carga/1 -> Subsystem/2(Iabc_L)
  Subsystem/1(Valpha') -> Subsystem1/1(Valpha'), Subsystem2/1(Valpha')
  Subsystem/3(Ialpha) -> Subsystem1/3(Ialpha)
  Subsystem/2(Vbeta') -> Subsystem1/2(Vbeta'), Subsystem2/2(Vbeta')
  Subsystem/4(Ibeta) -> Subsystem1/4(Ibeta)
  Subsystem1/1(Posc) -> Subsystem2/3(Posc)
  Subsystem1/2(q) -> Subsystem2/4(q)
  Subsystem3/1(Ia_C) -> Mux/1, Ia_C*/1
  Subsystem3/2(Ib_C) -> Mux/2, Ib_C*/1
  Subsystem3/3(Ic_C) -> Mux/3, Ic_C*/1
  Subsystem2/1(Ialpha_p) -> Subsystem3/1(Ialpha_p)
  Subsystem2/2(Ibeta_p) -> Subsystem3/2(Ibeta_p)
  Mux/1 -> To Workspace/1

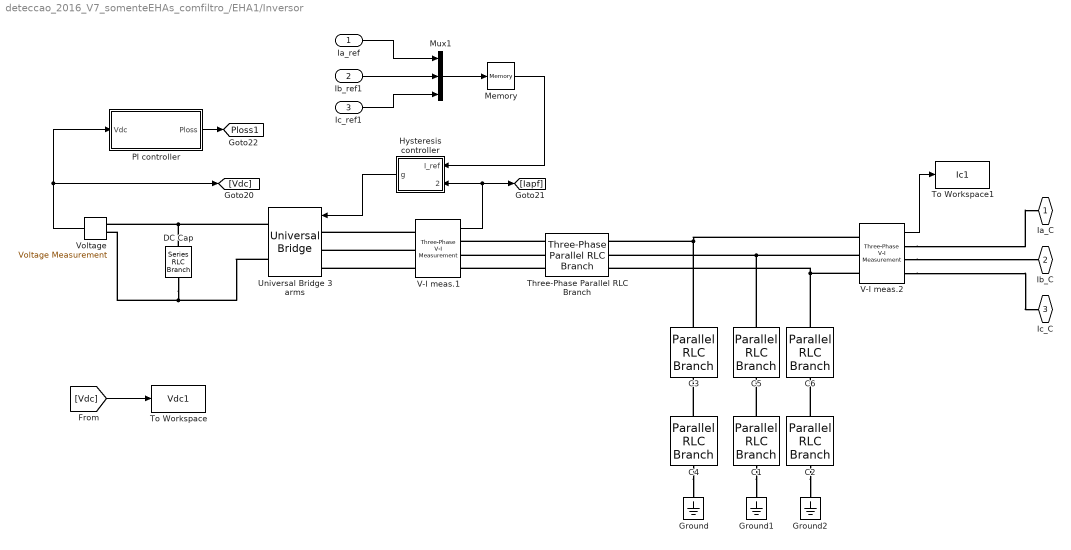
== system deteccao_2016_V7_somenteEHAs_comfiltro_/EHA1/Inversor ==
  Ia_ref : Inport
  Ib_ref1 : Inport  Port=2
  Ic_ref1 : Inport  Port=3
  C1 : powerlib/Elements/Parallel RLC Branch  LConnTagsString=a  RConnTagsString=__new0  BranchType=RC  Resistance=R2  Inductance=1e-3  SetiL0=off  InitialCurrent=0  Capacitance=C  Setx0=off  InitialVoltage=0  Measurements=None
  C2 : powerlib/Elements/Parallel RLC Branch  LConnTagsString=a  RConnTagsString=__new0  BranchType=RC  Resistance=R2  Inductance=1e-3  SetiL0=off  InitialCurrent=0  Capacitance=C  Setx0=off  InitialVoltage=0  Measurements=None
  C3 : powerlib/Elements/Parallel RLC Branch  LConnTagsString=a  RConnTagsString=__new0  BranchType=R  Resistance=R1  Inductance=1e-3  SetiL0=off  InitialCurrent=0  Capacitance=C  Setx0=off  InitialVoltage=0  Measurements=None
  C4 : powerlib/Elements/Parallel RLC Branch  LConnTagsString=a  RConnTagsString=__new0  BranchType=RC  Resistance=R2  Inductance=1e-3  SetiL0=off  InitialCurrent=0  Capacitance=C  Setx0=off  InitialVoltage=0  Measurements=None
  C5 : powerlib/Elements/Parallel RLC Branch  LConnTagsString=a  RConnTagsString=__new0  BranchType=R  Resistance=R1  Inductance=1e-3  SetiL0=off  InitialCurrent=0  Capacitance=C  Setx0=off  InitialVoltage=0  Measurements=None
  C6 : powerlib/Elements/Parallel RLC Branch  LConnTagsString=a  RConnTagsString=__new0  BranchType=R  Resistance=R1  Inductance=1e-3  SetiL0=off  InitialCurrent=0  Capacitance=C  Setx0=off  InitialVoltage=0  Measurements=None
  DC Cap : powerlib/Elements/Series RLC Branch  LConnTagsString=__new0  RConnTagsString=__new0  BranchType=C  Resistance=1  Inductance=1e-3  SetiL0=off  InitialCurrent=0  Capacitance=200e-6  Setx0=off  InitialVoltage=350  Measurements=None
  Ground : powerlib/Elements/Ground  LConnTagsString=a
  Ground1 : powerlib/Elements/Ground  LConnTagsString=a
  Ground2 : powerlib/Elements/Ground  LConnTagsString=a
  Hysteresis controller : Subsystem
  Memory : Memory
  Mux1 : Mux  Inputs=3
  PI controller : Subsystem
  Three-Phase Parallel RLC Branch : powerlib/Elements/Three-Phase Parallel RLC Branch  LConnTagsString=A|B|C  RConnTagsString=A|B|C  BranchType=L  Resistance=1  Inductance=L  Capacitance=1e-6  Measurements=None
  To Workspace : ToWorkspace  VariableName=Vdc1  SaveFormat=Structure With Time  SampleTime=-1
  To Workspace1 : ToWorkspace  VariableName=Ic1  SaveFormat=Structure With Time  SampleTime=-1
  Universal Bridge 3 arms : powerlib/Power Electronics/Universal Bridge  Arms=3  SnubberResistance=1e8  SnubberCapacitance=inf  Device=Ideal Switches  Ron=1e-5  Lon=0  ForwardVoltages="[  1  1  ]"  ForwardVoltage=.8  GTOparameters=[ 10e-6 , 20e-6 ]  IGBTparameters=[ 1e-6 , 2e-6 ]  Measurements=All voltages and currents  Measurements_2=None  converterType=Rectifier
  V-I meas.1 : powerlib/Measurements/Three-Phase V-I Measurement  VoltageMeasurement=no  SetLabelV=off  LabelV=Vnm_EHA1  Vpu=off  VpuLL=off  CurrentMeasurement=yes  SetLabelI=off  LabelI=Iabc  Ipu=off  Pbase=100e6  Vbase=500e3  OutputType=Complex  PhasorSimulation=off  PSBequivalent=0
  V-I meas.2 : powerlib/Measurements/Three-Phase V-I Measurement  VoltageMeasurement=no  SetLabelV=off  LabelV=Vnm_EHA1  Vpu=off  VpuLL=off  CurrentMeasurement=yes  SetLabelI=off  LabelI=Iabc  Ipu=off  Pbase=100e6  Vbase=500e3  OutputType=Complex  PhasorSimulation=off  PSBequivalent=0
  Voltage : powerlib/Measurements/Voltage Measurement  PhasorSimulation=off  OutputType=Complex  PSBequivalent=0
  Ia_C : PMIOPort  Port=1  Side=Right
  Ib_C : PMIOPort  Port=2  Side=Right
  Ic_C : PMIOPort  Port=3  Side=Right
  tag scope: Ploss1=global
  wires:
  Voltage/1 -> [Vdc], PI controller/1(Vdc)
  PI controller/1(Ploss) -> [Ploss1]
  V-I meas.1/1 -> Hysteresis controller/2(I_meas), [Iapf]
  Mux1/1 -> Memory/1
  Hysteresis controller/1(g) -> Universal Bridge 3 arms/1
  Ia_ref/1 -> Mux1/1
  Ib_ref1/1 -> Mux1/2
  Ic_ref1/1 -> Mux1/3
  Memory/1 -> Hysteresis controller/1(I_ref)
  [Vdc] -> To Workspace/1
  V-I meas.2/1 -> To Workspace1/1
  connections:
  Universal Bridge 3 arms/RConn1 -- DC Cap/LConn1 -- Voltage/LConn1
  Universal Bridge 3 arms/RConn2 -- DC Cap/RConn1 -- Voltage/LConn2
  Three-Phase Parallel RLC Branch/LConn2 -- V-I meas.1/RConn2
  V-I meas.1/LConn1 -- Universal Bridge 3 arms/LConn1
  Three-Phase Parallel RLC Branch/LConn1 -- V-I meas.1/RConn1
  V-I meas.1/LConn2 -- Universal Bridge 3 arms/LConn2
  Three-Phase Parallel RLC Branch/LConn3 -- V-I meas.1/RConn3
  V-I meas.1/LConn3 -- Universal Bridge 3 arms/LConn3
  V-I meas.2/RConn1 -- Ia_C/RConn1
  V-I meas.2/RConn2 -- Ib_C/RConn1
  V-I meas.2/RConn3 -- Ic_C/RConn1
  C4/RConn1 -- Ground/LConn1
  C1/RConn1 -- Ground1/LConn1
  C2/RConn1 -- Ground2/LConn1
  V-I meas.2/LConn1 -- C3/LConn1 -- Three-Phase Parallel RLC Branch/RConn1
  C1/LConn1 -- C5/RConn1
  V-I meas.2/LConn3 -- C6/LConn1 -- Three-Phase Parallel RLC Branch/RConn3
  C4/LConn1 -- C3/RConn1
  C5/LConn1 -- V-I meas.2/LConn2 -- Three-Phase Parallel RLC Branch/RConn2
  C2/LConn1 -- C6/RConn1

== system deteccao_2016_V7_somenteEHAs_comfiltro_/EHA1/Signal Builder ==
  Demux : Demux  Tag=STV Demux  Outputs=1
  FromWs : FromWorkspace  Tag=STV FromWs  VariableName=tuvar  SampleTime=0
      SigBuilderData=|
      | common.afterFinalStr = 'Extrapolate'
      | common.sampleTime = 0
      | dataSet.timeRange = [72.75 73.9]
      | dataSet.name = 'Imported_Group 1'
      | sbobj.Name = 'Signal Builder'
      | sbobj.Groups.Name = 'Imported_Group 1'
      | sbobj.Groups.Signals.Name = 'var'
      | sbobj.Groups.Signals.XData = [72.75 72.751 72.752 72.753 72.754 72.755 72.756 72.757 72.758 72.759 72.76 72.761 ... (1151 elements, 1x1151)]
      | sbobj.Groups.Signals.YData = [0 0 0 0 0 0 0 0 0 0 0 0 ... (1151 elements, 1x1151)]
      | sbobj.Groups.TimeRange = [72.75 73.9]
  var : Outport
  wires:
  Demux/1 -> var/1
  FromWs/1 -> Demux/1

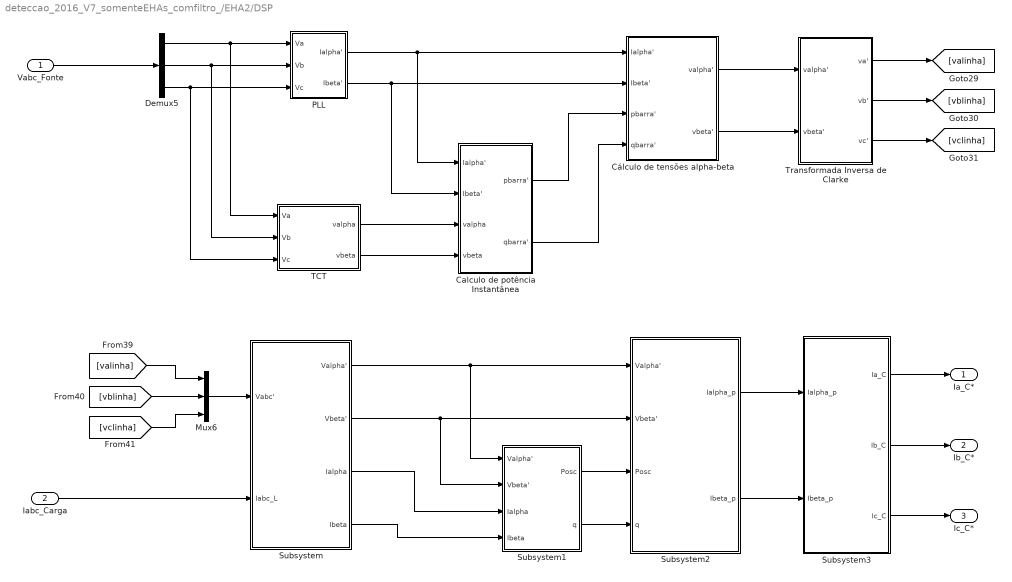
== system deteccao_2016_V7_somenteEHAs_comfiltro_/EHA2/DSP ==
  Vabc_Fonte : Inport
  Iabc_Carga : Inport  Port=2
  Calculo de potência Instantânea : Subsystem
  Cálculo de tensões alpha-beta : Subsystem
  Demux5 : Demux  Outputs=3
  Mux6 : Mux  Inputs=3
  PLL : Subsystem
  Subsystem : Subsystem
  Subsystem1 : Subsystem
  Subsystem2 : Subsystem
  Subsystem3 : Subsystem
  TCT : Subsystem
  Transformada Inversa de Clarke : Subsystem
  Ia_C* : Outport
  Ib_C* : Outport  Port=2
  Ic_C* : Outport  Port=3
  wires:
  Vabc_Fonte/1 -> Demux5/1
  Demux5/1 -> PLL/1(Va), TCT/1(Va)
  Demux5/2 -> PLL/2(Vb), TCT/2(Vb)
  Demux5/3 -> PLL/3(Vc), TCT/3(Vc)
  TCT/1(valpha) -> Calculo de potência Instantânea/3(valpha)
  TCT/2(vbeta) -> Calculo de potência Instantânea/4(vbeta)
  Calculo de potência Instantânea/2(qbarra') -> Cálculo de tensões alpha-beta/4(qbarra')
  PLL/1(Ialpha') -> Calculo de potência Instantânea/1(Ialpha'), Cálculo de tensões alpha-beta/1(Ialpha')
  PLL/2(Ibeta') -> Calculo de potência Instantânea/2(Ibeta'), Cálculo de tensões alpha-beta/2(Ibeta')
  Calculo de potência Instantânea/1(pbarra') -> Cálculo de tensões alpha-beta/3(pbarra')
  Cálculo de tensões alpha-beta/1(valpha') -> Transformada Inversa de Clarke/1(valpha')
  Cálculo de tensões alpha-beta/2(vbeta') -> Transformada Inversa de Clarke/2(vbeta')
  Transformada Inversa de Clarke/1(va') -> [valinha]
  Transformada Inversa de Clarke/2(vb') -> [vblinha]
  Transformada Inversa de Clarke/3(vc') -> [vclinha]
  [valinha] -> Mux6/1
  [vblinha] -> Mux6/2
  [vclinha] -> Mux6/3
  Mux6/1 -> Subsystem/1(Vabc')
  Iabc_Carga/1 -> Subsystem/2(Iabc_L)
  Subsystem/1(Valpha') -> Subsystem1/1(Valpha'), Subsystem2/1(Valpha')
  Subsystem/3(Ialpha) -> Subsystem1/3(Ialpha)
  Subsystem/2(Vbeta') -> Subsystem1/2(Vbeta'), Subsystem2/2(Vbeta')
  Subsystem/4(Ibeta) -> Subsystem1/4(Ibeta)
  Subsystem1/1(Posc) -> Subsystem2/3(Posc)
  Subsystem1/2(q) -> Subsystem2/4(q)
  Subsystem3/1(Ia_C) -> Ia_C*/1
  Subsystem3/2(Ib_C) -> Ib_C*/1
  Subsystem3/3(Ic_C) -> Ic_C*/1
  Subsystem2/1(Ialpha_p) -> Subsystem3/1(Ialpha_p)
  Subsystem2/2(Ibeta_p) -> Subsystem3/2(Ibeta_p)

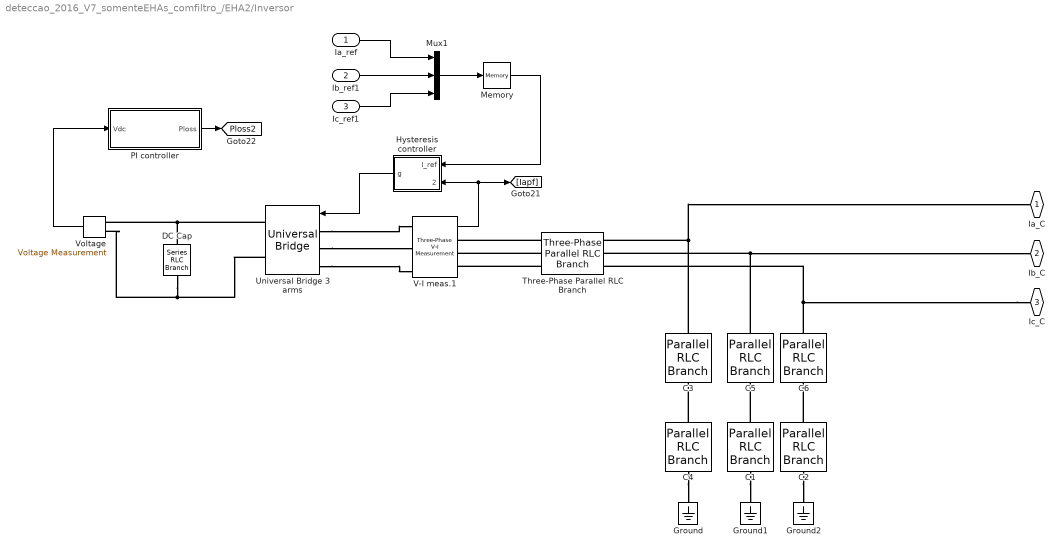
== system deteccao_2016_V7_somenteEHAs_comfiltro_/EHA2/Inversor ==
  Ia_ref : Inport
  Ib_ref1 : Inport  Port=2
  Ic_ref1 : Inport  Port=3
  C1 : powerlib/Elements/Parallel RLC Branch  LConnTagsString=a  RConnTagsString=__new0  BranchType=RC  Resistance=R2  Inductance=1e-3  SetiL0=off  InitialCurrent=0  Capacitance=C  Setx0=off  InitialVoltage=0  Measurements=None
  C2 : powerlib/Elements/Parallel RLC Branch  LConnTagsString=a  RConnTagsString=__new0  BranchType=RC  Resistance=R2  Inductance=1e-3  SetiL0=off  InitialCurrent=0  Capacitance=C  Setx0=off  InitialVoltage=0  Measurements=None
  C3 : powerlib/Elements/Parallel RLC Branch  LConnTagsString=a  RConnTagsString=__new0  BranchType=R  Resistance=R1  Inductance=1e-3  SetiL0=off  InitialCurrent=0  Capacitance=C  Setx0=off  InitialVoltage=0  Measurements=None
  C4 : powerlib/Elements/Parallel RLC Branch  LConnTagsString=a  RConnTagsString=__new0  BranchType=RC  Resistance=R2  Inductance=1e-3  SetiL0=off  InitialCurrent=0  Capacitance=C  Setx0=off  InitialVoltage=0  Measurements=None
  C5 : powerlib/Elements/Parallel RLC Branch  LConnTagsString=a  RConnTagsString=__new0  BranchType=R  Resistance=R1  Inductance=1e-3  SetiL0=off  InitialCurrent=0  Capacitance=C  Setx0=off  InitialVoltage=0  Measurements=None
  C6 : powerlib/Elements/Parallel RLC Branch  LConnTagsString=a  RConnTagsString=__new0  BranchType=R  Resistance=R1  Inductance=1e-3  SetiL0=off  InitialCurrent=0  Capacitance=C  Setx0=off  InitialVoltage=0  Measurements=None
  DC Cap : powerlib/Elements/Series RLC Branch  LConnTagsString=__new0  RConnTagsString=__new0  BranchType=C  Resistance=1  Inductance=1e-3  SetiL0=off  InitialCurrent=0  Capacitance=200e-6  Setx0=off  InitialVoltage=350  Measurements=None
  Ground : powerlib/Elements/Ground  LConnTagsString=a
  Ground1 : powerlib/Elements/Ground  LConnTagsString=a
  Ground2 : powerlib/Elements/Ground  LConnTagsString=a
  Hysteresis controller : Subsystem
  Memory : Memory
  Mux1 : Mux  Inputs=3
  PI controller : Subsystem
  Three-Phase Parallel RLC Branch : powerlib/Elements/Three-Phase Parallel RLC Branch  LConnTagsString=A|B|C  RConnTagsString=A|B|C  BranchType=L  Resistance=1  Inductance=L  Capacitance=1e-6  Measurements=None
  Universal Bridge 3 arms : powerlib/Power Electronics/Universal Bridge  Arms=3  SnubberResistance=1e8  SnubberCapacitance=inf  Device=Ideal Switches  Ron=1e-5  Lon=0  ForwardVoltages="[  1  1  ]"  ForwardVoltage=.8  GTOparameters=[ 10e-6 , 20e-6 ]  IGBTparameters=[ 1e-6 , 2e-6 ]  Measurements=None  Measurements_2=None  converterType=Rectifier
  V-I meas.1 : powerlib/Measurements/Three-Phase V-I Measurement  VoltageMeasurement=no  SetLabelV=off  LabelV=Vnm_EHA1  Vpu=off  VpuLL=off  CurrentMeasurement=yes  SetLabelI=off  LabelI=Iabc  Ipu=off  Pbase=100e6  Vbase=500e3  OutputType=Complex  PhasorSimulation=off  PSBequivalent=0
  Voltage : powerlib/Measurements/Voltage Measurement  PhasorSimulation=off  OutputType=Complex  PSBequivalent=0
  Ia_C : PMIOPort  Port=1  Side=Right
  Ib_C : PMIOPort  Port=2  Side=Right
  Ic_C : PMIOPort  Port=3  Side=Right
  tag scope: Ploss2=global
  wires:
  Voltage/1 -> PI controller/1(Vdc)
  PI controller/1(Ploss) -> [Ploss2]
  V-I meas.1/1 -> Hysteresis controller/2(I_meas), [Iapf]
  Mux1/1 -> Memory/1
  Hysteresis controller/1(g) -> Universal Bridge 3 arms/1
  Ia_ref/1 -> Mux1/1
  Ib_ref1/1 -> Mux1/2
  Ic_ref1/1 -> Mux1/3
  Memory/1 -> Hysteresis controller/1(I_ref)
  connections:
  Voltage/LConn1 -- Universal Bridge 3 arms/RConn1 -- DC Cap/LConn1
  Voltage/LConn2 -- Universal Bridge 3 arms/RConn2 -- DC Cap/RConn1
  Three-Phase Parallel RLC Branch/LConn2 -- V-I meas.1/RConn2
  Universal Bridge 3 arms/LConn1 -- V-I meas.1/LConn1
  Three-Phase Parallel RLC Branch/LConn1 -- V-I meas.1/RConn1
  Universal Bridge 3 arms/LConn2 -- V-I meas.1/LConn2
  Three-Phase Parallel RLC Branch/LConn3 -- V-I meas.1/RConn3
  Universal Bridge 3 arms/LConn3 -- V-I meas.1/LConn3
  Three-Phase Parallel RLC Branch/RConn1 -- C3/LConn1 -- Ia_C/RConn1
  Three-Phase Parallel RLC Branch/RConn2 -- C5/LConn1 -- Ib_C/RConn1
  Ic_C/RConn1 -- C6/LConn1 -- Three-Phase Parallel RLC Branch/RConn3
  C4/RConn1 -- Ground/LConn1
  C4/LConn1 -- C3/RConn1
  C2/LConn1 -- C6/RConn1
  C2/RConn1 -- Ground2/LConn1
  C1/LConn1 -- C5/RConn1
  C1/RConn1 -- Ground1/LConn1

== system deteccao_2016_V7_somenteEHAs_comfiltro_/EHA2/Signal Builder ==
  Demux : Demux  Tag=STV Demux  Outputs=1
  FromWs : FromWorkspace  Tag=STV FromWs  VariableName=tuvar  SampleTime=0
      SigBuilderData=|
      | common.afterFinalStr = 'Extrapolate'
      | common.sampleTime = 0
      | dataSet.timeRange = [72.75 73.9]
      | dataSet.name = 'Imported_Group 1'
      | sbobj.Name = 'Signal Builder'
      | sbobj.Groups.Name = 'Imported_Group 1'
      | sbobj.Groups.Signals.Name = 'var'
      | sbobj.Groups.Signals.XData = [72.75 72.751 72.752 72.753 72.754 72.755 72.756 72.757 72.758 72.759 72.76 72.761 ... (1151 elements, 1x1151)]
      | sbobj.Groups.Signals.YData = [0 0 0 0 0 0 0 0 0 0 0 0 ... (1151 elements, 1x1151)]
      | sbobj.Groups.TimeRange = [72.75 73.9]
  var : Outport
  wires:
  Demux/1 -> var/1
  FromWs/1 -> Demux/1

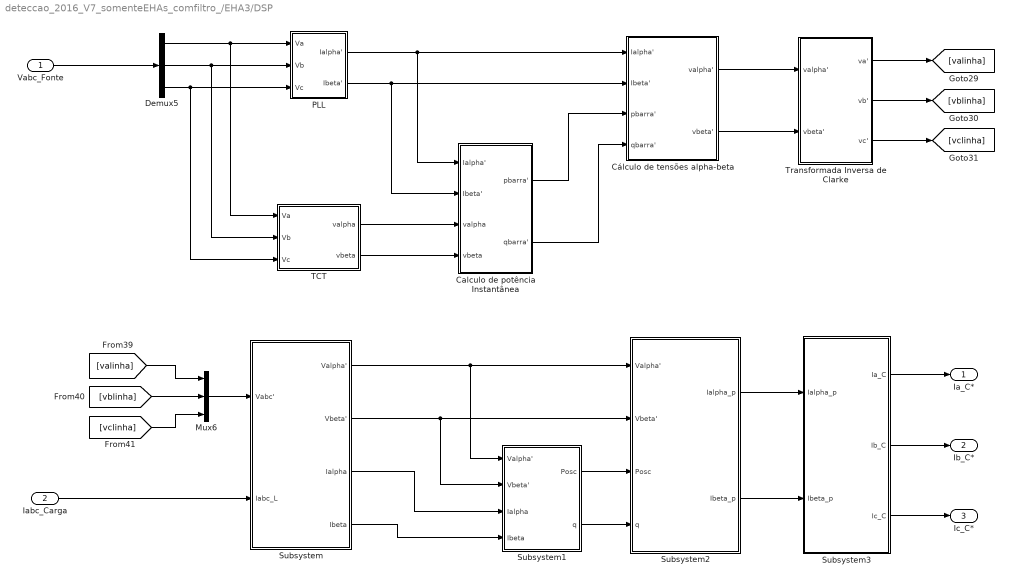
== system deteccao_2016_V7_somenteEHAs_comfiltro_/EHA3/DSP ==
  Vabc_Fonte : Inport
  Iabc_Carga : Inport  Port=2
  Calculo de potência Instantânea : Subsystem
  Cálculo de tensões alpha-beta : Subsystem
  Demux5 : Demux  Outputs=3
  Mux6 : Mux  Inputs=3
  PLL : Subsystem
  Subsystem : Subsystem
  Subsystem1 : Subsystem
  Subsystem2 : Subsystem
  Subsystem3 : Subsystem
  TCT : Subsystem
  Transformada Inversa de Clarke : Subsystem
  Ia_C* : Outport
  Ib_C* : Outport  Port=2
  Ic_C* : Outport  Port=3
  wires:
  Vabc_Fonte/1 -> Demux5/1
  Demux5/1 -> PLL/1(Va), TCT/1(Va)
  Demux5/2 -> PLL/2(Vb), TCT/2(Vb)
  Demux5/3 -> PLL/3(Vc), TCT/3(Vc)
  TCT/1(valpha) -> Calculo de potência Instantânea/3(valpha)
  TCT/2(vbeta) -> Calculo de potência Instantânea/4(vbeta)
  Calculo de potência Instantânea/2(qbarra') -> Cálculo de tensões alpha-beta/4(qbarra')
  PLL/1(Ialpha') -> Calculo de potência Instantânea/1(Ialpha'), Cálculo de tensões alpha-beta/1(Ialpha')
  PLL/2(Ibeta') -> Calculo de potência Instantânea/2(Ibeta'), Cálculo de tensões alpha-beta/2(Ibeta')
  Calculo de potência Instantânea/1(pbarra') -> Cálculo de tensões alpha-beta/3(pbarra')
  Cálculo de tensões alpha-beta/1(valpha') -> Transformada Inversa de Clarke/1(valpha')
  Cálculo de tensões alpha-beta/2(vbeta') -> Transformada Inversa de Clarke/2(vbeta')
  Transformada Inversa de Clarke/1(va') -> [valinha]
  Transformada Inversa de Clarke/2(vb') -> [vblinha]
  Transformada Inversa de Clarke/3(vc') -> [vclinha]
  [valinha] -> Mux6/1
  [vblinha] -> Mux6/2
  [vclinha] -> Mux6/3
  Mux6/1 -> Subsystem/1(Vabc')
  Iabc_Carga/1 -> Subsystem/2(Iabc_L)
  Subsystem/1(Valpha') -> Subsystem1/1(Valpha'), Subsystem2/1(Valpha')
  Subsystem/3(Ialpha) -> Subsystem1/3(Ialpha)
  Subsystem/2(Vbeta') -> Subsystem1/2(Vbeta'), Subsystem2/2(Vbeta')
  Subsystem/4(Ibeta) -> Subsystem1/4(Ibeta)
  Subsystem1/1(Posc) -> Subsystem2/3(Posc)
  Subsystem1/2(q) -> Subsystem2/4(q)
  Subsystem3/1(Ia_C) -> Ia_C*/1
  Subsystem3/2(Ib_C) -> Ib_C*/1
  Subsystem3/3(Ic_C) -> Ic_C*/1
  Subsystem2/1(Ialpha_p) -> Subsystem3/1(Ialpha_p)
  Subsystem2/2(Ibeta_p) -> Subsystem3/2(Ibeta_p)
